simulink model "vexv5_Clawbot_MATLAB_Auto_Sequential"  (R2019a)
settings: Solver=ode3  StartTime=0.0  StopTime=inf  RelTol=1e-3  EnableMultiTasking=on
libraries: vexv5lib x4
settings Model: ExtModeTrigDuration=5  Creator=The MathWorks, Inc.  LastModifiedBy=josea
settings DataIOCC: LimitDataPoints=on  SaveFormat=Array  ReturnWorkspaceOutputs=off
settings OptimizationCC: ExpressionDepthLimit=2147483647  LifeSpan=Inf  MaxStackSize=64
settings DebuggingCC: UnderspecifiedInitializationDetection=Classic  MergeDetectMultiDrivingBlocksExec=none  InheritedTsInSrcMsg=none  FcnCallInpInsideContextMsg=warning  UnconnectedInputMsg=none  UnconnectedOutputMsg=none  AllowSymbolicDim=off  StateNameClashWarn=warning  SFUnexpectedBacktrackingDiag=warning  SFNoUnconditionalDefaultTransitionDiag=warning  SFExecutionAtInitializationDiag=none  ArithmeticOperatorsInVariantConditions=warning
settings HardwareCC: ProdBitPerPointer=32  ProdBitPerSizeT=32  ProdBitPerPtrDiffT=32  ProdLargestAtomicInteger=Long  ProdLargestAtomicFloat=Double  ProdWordSize=32  ProdHWDeviceType=ARM Compatible->ARM Cortex
settings ModelReferenceCC: PropagateSignalLabelsOutOfModel=off
settings SFSimCC: SimUseLocalCustomCode=off
settings RTWCC: SystemTargetFile=ert.tlc  HardwareBoard=VEX V5 Robot Brain  TLCOptions=-aInlineSetEventsForThisBaseRateFcn=TLC_FALSE -aSuppressMultiTaskScheduler=TLC_FALSE -aRateBasedStepFcn=0  TemplateMakefile=ert_default_tmf  RTWUseLocalCustomCode=off  Toolchain=GNU Tools for ARM Embedded Processors
settings CodeAppCC: StateflowObjectComments=on
settings ERTTargetCC: CodeReplacementLibrary=GCC ARM Cortex-M3  MultiwordLength=2048  ERTCustomFileBanners=off  SupportContinuousTime=on  SupportNonInlinedSFcns=on  RemoveResetFunc=off  ModelStepFunctionPrototypeControlCompliant=off  ConvertIfToSwitch=off  SuppressUnreachableDefaultCases=off
settings ConfigComp: CovMetricSettings=dw  CovHtmlReporting=on  CovSaveCumulativeToWorkspaceVar=on  CovSaveSingleToWorkspaceVar=on  CovExternalEMLEnable=off  CovSFcnEnable=off

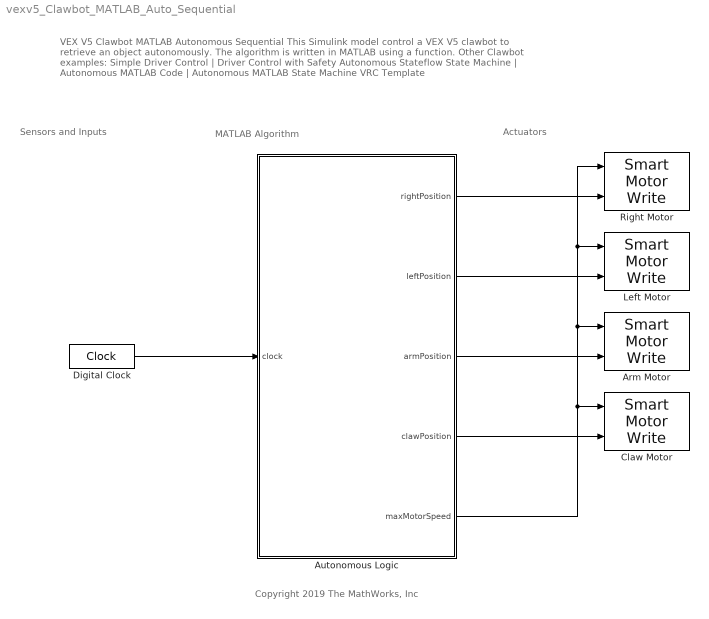
== system vexv5_Clawbot_MATLAB_Auto_Sequential ==
  note: Actuators
  note: MATLAB Algorithm
  note: Sensors and Inputs
  note: Copyright 2019 The MathWorks, Inc
  note: VEX V5 Clawbot MATLAB Autonomous Sequential
      | This Simulink model control a VEX V5 clawbot to retrieve an object autonomously.
      | The algorithm is written in MATLAB using a function. Other Clawbot examples:
      | Simple Driver Control | Driver Control with Safety
      | Autonomous Stateflow State Machine | Autonomous MATLAB Code | Autonomous MATLAB State Machine
      | VRC Template
  Arm Motor : vexv5lib/Actuators/Smart Motor Write  motorPort=8  scaleFactor=18:1  MotorBrakeMode=Brake  OperationMode=Position Control
      settings: SourceProductName=Simulink Coder Support Package for VEX EDR V5 Robot Brain
  Autonomous Logic : MATLAB Function  TreatAsAtomicUnit=on
  Claw Motor : vexv5lib/Actuators/Smart Motor Write  motorPort=3  scaleFactor=18:1  MotorBrakeMode=Brake  OperationMode=Position Control
      settings: SourceProductName=Simulink Coder Support Package for VEX EDR V5 Robot Brain
  Digital Clock : DigitalClock  SampleTime=0.05
  Left Motor : vexv5lib/Actuators/Smart Motor Write  motorPort=1  scaleFactor=18:1  MotorBrakeMode=Brake  OperationMode=Position Control
      settings: SourceProductName=Simulink Coder Support Package for VEX EDR V5 Robot Brain
  Right Motor : vexv5lib/Actuators/Smart Motor Write  motorPort=10  scaleFactor=18:1  MotorBrakeMode=Brake  OperationMode=Position Control
      settings: SourceProductName=Simulink Coder Support Package for VEX EDR V5 Robot Brain
  wires:
  Digital Clock/1 -> Autonomous Logic/1(clock)
  Autonomous Logic/5(maxMotorSpeed) -> Right Motor/1, Left Motor/1, Arm Motor/1, Claw Motor/1
  Autonomous Logic/1(rightPosition) -> Right Motor/2
  Autonomous Logic/2(leftPosition) -> Left Motor/2
  Autonomous Logic/3(armPosition) -> Arm Motor/2
  Autonomous Logic/4(clawPosition) -> Claw Motor/2

== matlab function vexv5_Clawbot_MATLAB_Auto_Sequential/Autonomous Logic ==
  data: rightPosition output; leftPosition output; armPosition output; clawPosition output; maxMotorSpeed output; clock input
function [rightPosition,leftPosition,armPosition,clawPosition,maxMotorSpeed] = robotControl(clock)
% This MATLAB function contains the logic to have a VEX clawbot
% navigate to automatically fetch and object based on timed motor commands

%% Variable Initialization
% Persistent variables allow values to be stored within the MATLAB function
% making them available for the algorithm regardless of the time step
persistent rightRotations leftRotations clawState armState
maxMotorSpeed=40;
 
% This portion of code initializes any persistent variables to a desired
% value
if isempty(leftRotations)
    rightRotations = 0;
    leftRotations = 0;
    clawState = 0;
    armState = 0;
end

%% Sequence of commands corresponding to periods of time

if clock < 4
    % Open Claw and Move Forward for first 4 seconds
    clawState = -480;
    rightRotations = -1800;
    leftRotations = 1800; 
elseif clock > 4 && clock < 5
    % Close Claw (4-5 seconds)
    clawState = 0;
elseif clock > 5 && clock < 6
    % Lift Arm (5-6 seconds)
    armState = 800;
elseif clock > 6 && clock < 10
    % Turn around (6-10 seconds)
    rightRotations = -3150;
    leftRotations = 450;
elseif clock >10 && clock < 14
    % Move forward again (10-14 seconds)
    rightRotations = -4950;
    leftRotations = 2250;
elseif clock >14
    % Open Claw and lower Arm
    clawState = -480;
    armState = 0;  
end

rightPosition = rightRotations;
leftPosition = leftRotations;
clawPosition = clawState;
armPosition = armState;
